simulink model "Simulink_pendulo"  (R2021a)
settings: Solver=VariableStepAuto  StartTime=0.0  StopTime=7  RelTol=1e-3
values from neighbouring files (symbols this model uses):
  Ts = mean(diff(t))    [identificacion_tfest.m]
libraries: cstblocks x3
settings Model: Creator=Pedro  LastModifiedBy=Pedro

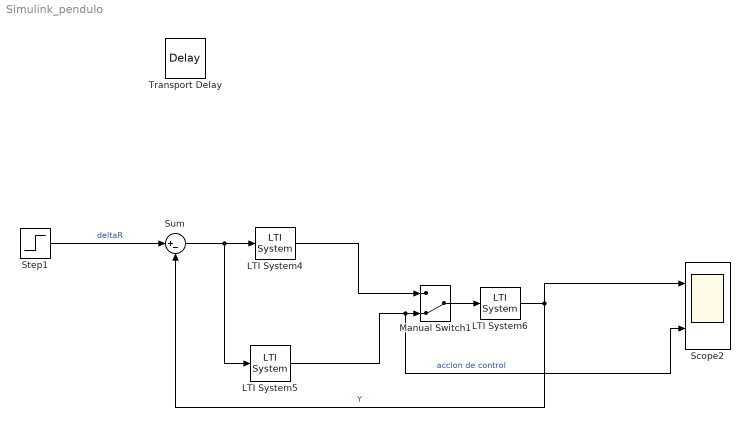
== system Simulink_pendulo ==
  LTI System4 : cstblocks/LTI System  sys=C_prop  IC=[]
  LTI System5 : cstblocks/LTI System  sys=C_PI  IC=[]
  LTI System6 : cstblocks/LTI System  sys=P  IC=[]
  Manual Switch1 : ManualSwitch  CurrentSetting=0
  Scope2 : Scope  NumInputPorts=2
  Step1 : Step  After=0.5  SampleTime=0
  Sum : Sum  Inputs=|+-
  Transport Delay : TransportDelay  DelayTime=Ts/4
  wires:
  LTI System6/1 -> Sum/2, Scope2/1  "Y"
  Sum/1 -> LTI System5/1, LTI System4/1
  Manual Switch1/1 -> LTI System6/1
  LTI System5/1 -> Scope2/2, Manual Switch1/2  "accion de control"
  Step1/1 -> Sum/1  "deltaR"
  LTI System4/1 -> Manual Switch1/1
